simulink model "OUT7"  (R2018a)
settings: Solver=VariableStepAuto  StartTime=0.0  StopTime=10.0  RelTol=1e-3
settings Model: Creator=Home  LastModifiedBy=Home

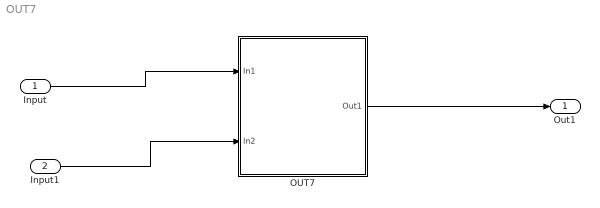
== system OUT7 ==
  Input : Inport
  Input1 : Inport  Port=2
  OUT7 : Subsystem
  Out1 : Outport
  wires:
  Input/1 -> OUT7/1(In1)
  Input1/1 -> OUT7/2(In2)
  OUT7/1(Out1) -> Out1/1

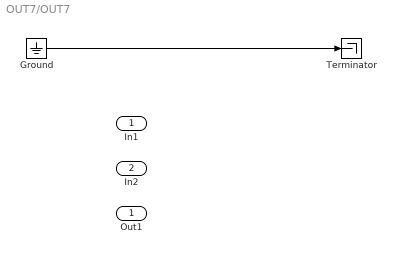
== system OUT7/OUT7 ==
  In1 : Inport
  In2 : Inport  Port=2
  Ground : Ground
  Terminator : Terminator
  Out1 : Outport
  wires:
  Ground/1 -> Terminator/1
